simulink model "estimator"  (R2016b)
settings: Solver=VariableStepAuto  StartTime=0.0  StopTime=10.0  RelTol=1e-3
settings Model: Creator=Anass  LastModifiedBy=Anass

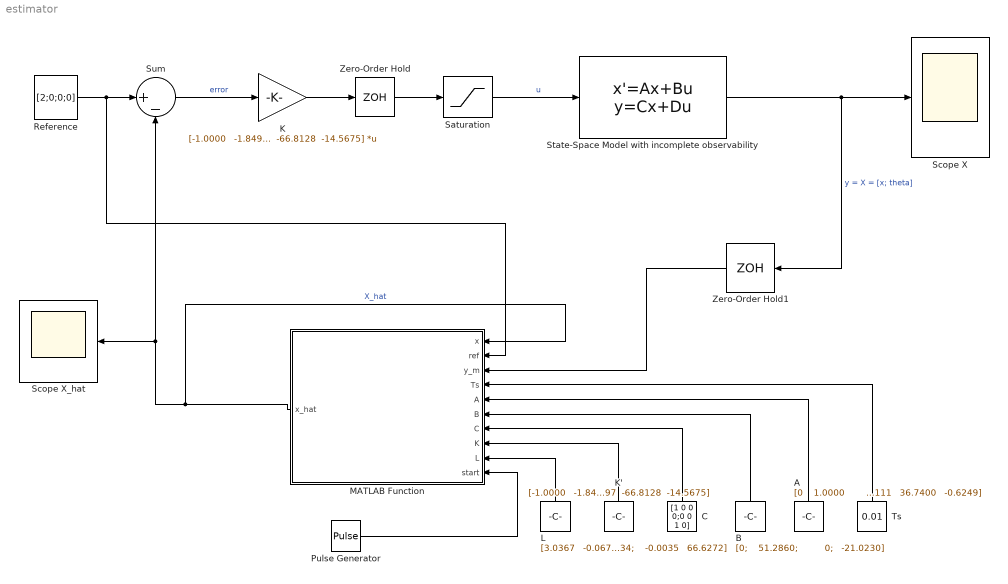
== system estimator ==
  A : Constant  Value=|
      | [0    1.0000         0         0;
      |          0  -10.4100         0         0;
      |          0         0         0    1.0000;
      |          0    4.3111   36.7400   -0.6249]
  B : Constant  Value=|
      | [0;
      |    51.2860;
      |          0;
      |   -21.0230]
  C : Constant  Value=[1 0 0 0;0 0 1 0]
  K : Gain  Gain="[-1.0000   -1.8497  -66.8128  -14.5675]"  Multiplication=Matrix(K*u) (u vector)
  K' : Constant  Value="[-1.0000   -1.8497  -66.8128  -14.5675]"
  L : Constant  Value=|
      | [3.0367   -0.0678;
      |     4.6131   -0.9845;
      |    -0.0678   11.5434;
      |    -0.0035   66.6272]
  MATLAB Function : MATLAB Function  TreatAsAtomicUnit=on
  Pulse Generator : DiscretePulseGenerator  PulseType=Time based  Period=50  PulseWidth=90  PhaseDelay=0.01
  Reference : Constant  Value=[2;0;0;0]
  Saturation : Saturate  UpperLimit=0.9  LowerLimit=-0.8
  Scope X : Scope
  Scope X_hat : Scope
  State-Space Model with incomplete observability : StateSpace  A=|  B=|  C=[1 0 0 0;0 0 1 0]  D=[0; 0]  X0=[1; 0; 0.1; 0]
      A=|
      | [0    1.0000         0         0;
      |          0  -10.4100         0         0;
      |          0         0         0    1.0000;
      |          0    4.3111   36.7400   -0.6249]
      B=|
      | [0;
      |    51.2860;
      |          0;
      |   -21.0230]
  Sum : Sum  Inputs=|+-
  Ts : Constant  Value=0.01
  Zero-Order Hold : ZeroOrderHold  SampleTime=0.01
  Zero-Order Hold1 : ZeroOrderHold  SampleTime=0.01
  wires:
  State-Space Model with incomplete observability/1 -> Zero-Order Hold1/1, Scope X/1  "y = X = [x; theta]"
  Sum/1 -> K/1  "error"
  Reference/1 -> MATLAB Function/2(ref), Sum/1
  K/1 -> Zero-Order Hold/1
  Zero-Order Hold/1 -> Saturation/1
  MATLAB Function/1(x_hat) -> MATLAB Function/1(x), Sum/2, Scope X_hat/1  "X_hat"
  Saturation/1 -> State-Space Model with incomplete observability/1  "u"
  Zero-Order Hold1/1 -> MATLAB Function/3(y_m)
  Ts/1 -> MATLAB Function/4(Ts)
  A/1 -> MATLAB Function/5(A)
  B/1 -> MATLAB Function/6(B)
  C/1 -> MATLAB Function/7(C)
  K'/1 -> MATLAB Function/8(K)
  L/1 -> MATLAB Function/9(L)
  Pulse Generator/1 -> MATLAB Function/10(start)

== matlab function estimator/MATLAB Function ==
  settings: updateMethod=DISCRETE  sampleTime=0.01
  data: x input; ref input; y_m input; x_hat output; Ts input; A input; B input; C input; K input; L input; start input
function x_hat = estimator(x,ref,y_m,Ts, A, B, C, K, L,start)
x_ini = [y_m(1); 0;  y_m(2); 0];
if start
    error_estimation = y_m - C*x_ini; % error of the estimation
    states = Ts*(A-B*K+eye(4))*x_ini + Ts*B*K*ref + Ts*L*error_estimation; % x_hat
else
    error_estimation = y_m - C*x; % error of the estimation
    states = Ts*(A-B*K+eye(4))*x + Ts*B*K*ref + Ts*L*error_estimation; % x_hat
end
x_hat = states;
end
